simulink model "Power_system_RZA_tau"  (R2017a)
settings: Solver=ode45  StartTime=0.0  StopTime=150  MaxStep=1e-4  RelTol=1e-3
values from neighbouring files (symbols this model uses):
  A2 = [0 1;0 0]    [Power_system_RZA_m.m]
  alpha = [alpha1;alpha0]    [Power_system_RZA_m.m]
  alpha0 = 1    [Power_system_RZA_m.m]
  B2 = [0;1]    [Power_system_RZA_m.m]
  C2 = [1 0]    [Power_system_RZA_m.m]
  Delta_f0 = 0    [Power_system_RZA_m.m]
  Delta_P0 = 0    [Power_system_RZA_m.m]
  Delta_X0 = 0.011    [Power_system_RZA_m.m]
  denC = conv([1 0],[tauC 1])    [Power_system_RZA_m.m]
  gn = -2*Klm/Tlm/Tg    (= -1.66666666667)    [Power_system_RZA_m.m]
  Gn = 3/Thn/Klm*(-1-Tlm/Thn)    (= -1.875)    [Power_system_RZA_m.m]
  Klm = 1    [Power_system_RZA_m.m]
  ks = -10    [Power_system_RZA_m.m]
  numC = [1.8124 -18.8558 0.1523]    [Power_system_RZA_m.m]
  ooverline_sat = overline_sat -1/ks    (= 20000.1)    [Power_system_RZA_m.m]
  overline_phin = [phin2; phin1]    [Power_system_RZA_m.m]
  overline_sat = 20000    [Power_system_RZA_m.m]
  psin = Klm/Tlm/Thn + Klm/Tlm/Tg    (= 0.875)    [Power_system_RZA_m.m]
  R = 0.05    [Power_system_RZA_m.m]
  Sn = 1/Thn    (= 0.25)    [Power_system_RZA_m.m]
  tau = 0.001    [Power_system_RZA_m.m]
  tau1 = 0.05    [Power_system_RZA_m.m]
  tau2 = 0.005    [Power_system_RZA_m.m]
  tau3 = 0.001    [Power_system_RZA_m.m]
  Tg = 0.2    [Power_system_RZA_m.m]
  Th2 = 6    [Power_system_RZA_m.m]
  Tlm = 6    [Power_system_RZA_m.m]
  ttrig = 60    [Power_system_RZA_m.m]
  underline_Delta1 = [tau1 0;0 tau1^2]    [Power_system_RZA_m.m]
  underline_Delta2 = [tau2 0;0 tau2^2]    [Power_system_RZA_m.m]
  underline_Delta3 = [tau3 0;0 tau3^2]    [Power_system_RZA_m.m]
  uunderline_sat = underline_sat + 1/ks    (= -20000.1)    [Power_system_RZA_m.m]
  zna0 = -0.001    [Power_system_RZA_m.m]
settings Model: Creator=Gyunghoon  LastModifiedBy=Gyunghoon
settings DataIOCC: LimitDataPoints=on  SaveFormat=Array
settings OptimizationCC: BlockReduction=off  BooleanDataType=off  LifeSpan=inf
settings DebuggingCC: SaveWithParameterizedLinksMsg=none  UnderspecifiedInitializationDetection=Classic  MergeDetectMultiDrivingBlocksExec=none  SignalResolutionControl=TryResolveAllWithWarning  SFUnexpectedBacktrackingDiag=warning  SFNoUnconditionalDefaultTransitionDiag=warning  SFExecutionAtInitializationDiag=none
settings HardwareCC: ProdBitPerPointer=32  ProdBitPerSizeT=32  ProdBitPerPtrDiffT=32  ProdLargestAtomicFloat=None  ProdIntDivRoundTo=Undefined  ProdEndianess=Unspecified  ProdWordSize=32  ProdHWDeviceType=32-bit Generic  TargetUnknown=on
settings ModelReferenceCC: PropagateSignalLabelsOutOfModel=off
settings GRTTargetCC: TargetLangStandard=C89/C90 (ANSI)  GeneratePreprocessorConditionals=Disable all
settings ConfigComp: CovMetricSettings=dw  CovHtmlReporting=on  CovSaveCumulativeToWorkspaceVar=on  CovSaveSingleToWorkspaceVar=on  CovExternalEMLEnable=off  CovSFcnEnable=off

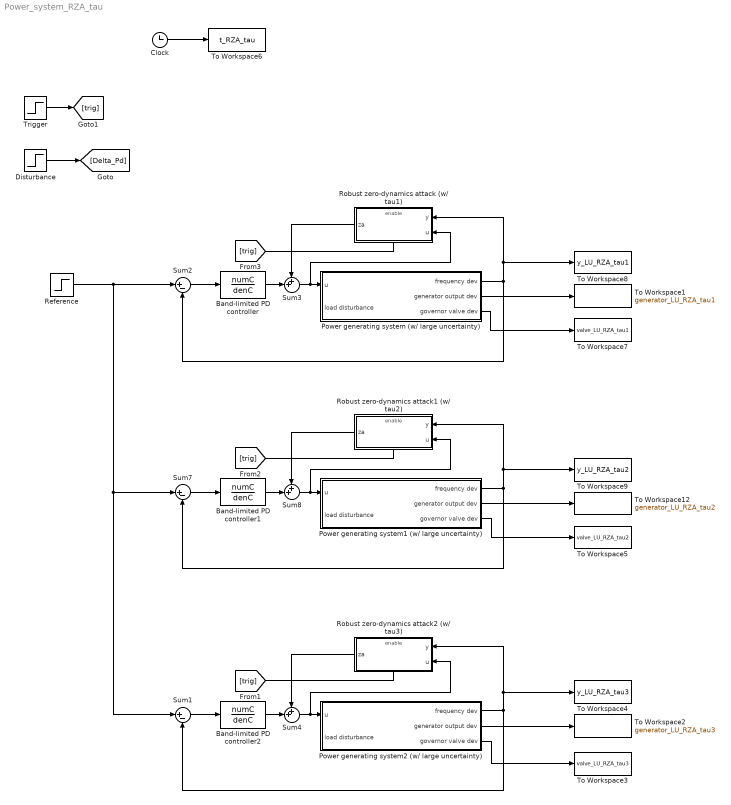
== system Power_system_RZA_tau ==
  Band-limited PD controller : TransferFcn  Numerator=numC  Denominator=denC
  Band-limited PD controller1 : TransferFcn  Numerator=numC  Denominator=denC
  Band-limited PD controller2 : TransferFcn  Numerator=numC  Denominator=denC
  Clock : Clock
  Disturbance : Step  Time=0  After=0.01  SampleTime=0
  Power generating system (w/ large uncertainty) : Subsystem
  Power generating system1 (w/ large uncertainty) : Subsystem
  Power generating system2 (w/ large uncertainty) : Subsystem
  Reference : Step  Time=0  After=0  SampleTime=0
  Robust zero-dynamics attack (w/ tau1) : Subsystem  TreatAsAtomicUnit=on
  Robust zero-dynamics attack1 (w/ tau2) : Subsystem  TreatAsAtomicUnit=on
  Robust zero-dynamics attack2 (w/ tau3) : Subsystem  TreatAsAtomicUnit=on
  Sum1 : Sum  Inputs=|+-
  Sum2 : Sum  Inputs=|+-
  Sum3 : Sum  Inputs=++|
  Sum4 : Sum  Inputs=++|
  Sum7 : Sum  Inputs=|+-
  Sum8 : Sum  Inputs=++|
  To Workspace1 : ToWorkspace  VariableName=generator_LU_RZA_tau1  SampleTime=-1
  To Workspace12 : ToWorkspace  VariableName=generator_LU_RZA_tau2  SampleTime=-1
  To Workspace2 : ToWorkspace  VariableName=generator_LU_RZA_tau3  SampleTime=-1
  To Workspace3 : ToWorkspace  VariableName=valve_LU_RZA_tau3  SampleTime=-1
  To Workspace4 : ToWorkspace  VariableName=y_LU_RZA_tau3  SampleTime=-1
  To Workspace5 : ToWorkspace  VariableName=valve_LU_RZA_tau2  SampleTime=-1
  To Workspace6 : ToWorkspace  VariableName=t_RZA_tau  SampleTime=-1
  To Workspace7 : ToWorkspace  VariableName=valve_LU_RZA_tau1  SampleTime=-1
  To Workspace8 : ToWorkspace  VariableName=y_LU_RZA_tau1  SampleTime=-1
  To Workspace9 : ToWorkspace  VariableName=y_LU_RZA_tau2  SampleTime=-1
  Trigger : Step  Time=ttrig  SampleTime=0
  wires:
  Disturbance/1 -> [Delta_Pd]
  Sum7/1 -> Band-limited PD controller1/1
  Band-limited PD controller1/1 -> Sum8/2
  Power generating system1 (w/ large uncertainty)/3(governor valve dev) -> To Workspace5/1
  Clock/1 -> To Workspace6/1
  Power generating system1 (w/ large uncertainty)/1(frequency dev) -> To Workspace9/1, Robust zero-dynamics attack1 (w/ tau2)/1(y), Sum7/2
  Sum8/1 -> Robust zero-dynamics attack1 (w/ tau2)/2(u), Power generating system1 (w/ large uncertainty)/1(u)
  Robust zero-dynamics attack1 (w/ tau2)/1(za) -> Sum8/1
  Trigger/1 -> [trig]
  [trig] -> Robust zero-dynamics attack1 (w/ tau2)/Enable
  Power generating system1 (w/ large uncertainty)/2(generator output dev) -> To Workspace12/1
  Sum1/1 -> Band-limited PD controller2/1
  Band-limited PD controller2/1 -> Sum4/2
  Power generating system2 (w/ large uncertainty)/3(governor valve dev) -> To Workspace3/1
  Power generating system2 (w/ large uncertainty)/1(frequency dev) -> To Workspace4/1, Robust zero-dynamics attack2 (w/ tau3)/1(y), Sum1/2
  Sum4/1 -> Robust zero-dynamics attack2 (w/ tau3)/2(u), Power generating system2 (w/ large uncertainty)/1(u)
  Robust zero-dynamics attack2 (w/ tau3)/1(za) -> Sum4/1
  [trig] -> Robust zero-dynamics attack2 (w/ tau3)/Enable
  Power generating system2 (w/ large uncertainty)/2(generator output dev) -> To Workspace2/1
  Sum2/1 -> Band-limited PD controller/1
  Reference/1 -> Sum1/1, Sum7/1, Sum2/1
  Band-limited PD controller/1 -> Sum3/2
  Power generating system (w/ large uncertainty)/3(governor valve dev) -> To Workspace7/1
  Power generating system (w/ large uncertainty)/1(frequency dev) -> To Workspace8/1, Robust zero-dynamics attack (w/ tau1)/1(y), Sum2/2
  Sum3/1 -> Robust zero-dynamics attack (w/ tau1)/2(u), Power generating system (w/ large uncertainty)/1(u)
  Robust zero-dynamics attack (w/ tau1)/1(za) -> Sum3/1
  [trig] -> Robust zero-dynamics attack (w/ tau1)/Enable
  Power generating system (w/ large uncertainty)/2(generator output dev) -> To Workspace1/1

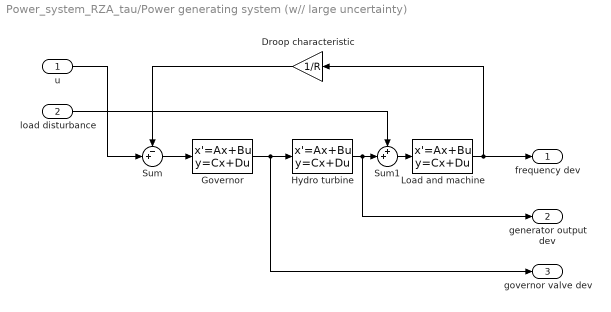
== system Power_system_RZA_tau/Power generating system (w// large uncertainty) ==
  u : Inport
  load disturbance : Inport  Port=2
  Droop characteristic : Gain  Gain=1/R
  Governor : StateSpace  A=-1/Tg  B=1/Tg  D=0  X0=Delta_X0
  Hydro turbine : StateSpace  A=-2/Th2  B=6/Th2  D=-2  X0=Delta_P0+2*Delta_X0
  Load and machine : StateSpace  A=-1/Tlm  B=Klm/Tlm  D=0  X0=Delta_f0
  Sum : Sum  Inputs=-+|
  Sum1 : Sum  Inputs=++|
  frequency dev : Outport
  generator output dev : Outport  Port=2
  governor valve dev : Outport  Port=3
  wires:
  u/1 -> Sum/2
  Droop characteristic/1 -> Sum/1
  Load and machine/1 -> Droop characteristic/1, frequency dev/1
  Hydro turbine/1 -> generator output dev/1, Sum1/2
  Sum/1 -> Governor/1
  Governor/1 -> Hydro turbine/1, governor valve dev/1
  Sum1/1 -> Load and machine/1
  load disturbance/1 -> Sum1/1

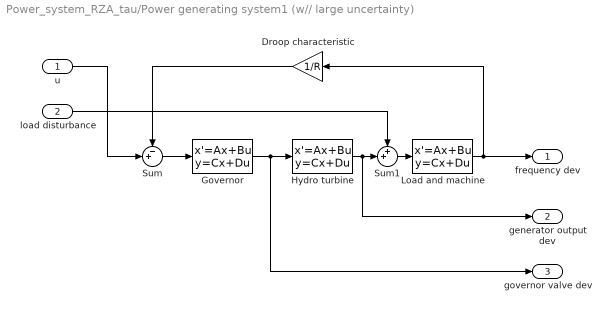
== system Power_system_RZA_tau/Power generating system1 (w// large uncertainty) ==
  u : Inport
  load disturbance : Inport  Port=2
  Droop characteristic : Gain  Gain=1/R
  Governor : StateSpace  A=-1/Tg  B=1/Tg  D=0  X0=Delta_X0
  Hydro turbine : StateSpace  A=-2/Th2  B=6/Th2  D=-2  X0=Delta_P0+2*Delta_X0
  Load and machine : StateSpace  A=-1/Tlm  B=Klm/Tlm  D=0  X0=Delta_f0
  Sum : Sum  Inputs=-+|
  Sum1 : Sum  Inputs=++|
  frequency dev : Outport
  generator output dev : Outport  Port=2
  governor valve dev : Outport  Port=3
  wires:
  u/1 -> Sum/2
  Droop characteristic/1 -> Sum/1
  Load and machine/1 -> Droop characteristic/1, frequency dev/1
  Hydro turbine/1 -> generator output dev/1, Sum1/2
  Sum/1 -> Governor/1
  Governor/1 -> Hydro turbine/1, governor valve dev/1
  Sum1/1 -> Load and machine/1
  load disturbance/1 -> Sum1/1

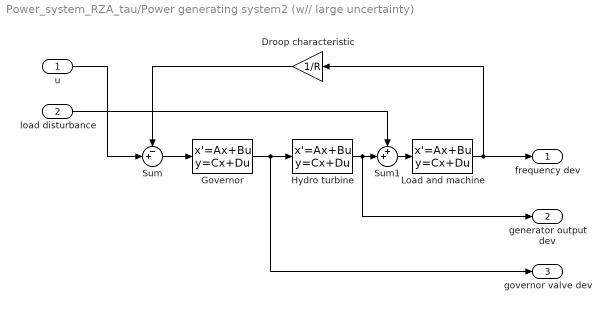
== system Power_system_RZA_tau/Power generating system2 (w// large uncertainty) ==
  u : Inport
  load disturbance : Inport  Port=2
  Droop characteristic : Gain  Gain=1/R
  Governor : StateSpace  A=-1/Tg  B=1/Tg  D=0  X0=Delta_X0
  Hydro turbine : StateSpace  A=-2/Th2  B=6/Th2  D=-2  X0=Delta_P0+2*Delta_X0
  Load and machine : StateSpace  A=-1/Tlm  B=Klm/Tlm  D=0  X0=Delta_f0
  Sum : Sum  Inputs=-+|
  Sum1 : Sum  Inputs=++|
  frequency dev : Outport
  generator output dev : Outport  Port=2
  governor valve dev : Outport  Port=3
  wires:
  u/1 -> Sum/2
  Droop characteristic/1 -> Sum/1
  Load and machine/1 -> Droop characteristic/1, frequency dev/1
  Hydro turbine/1 -> generator output dev/1, Sum1/2
  Sum/1 -> Governor/1
  Governor/1 -> Hydro turbine/1, governor valve dev/1
  Sum1/1 -> Load and machine/1
  load disturbance/1 -> Sum1/1

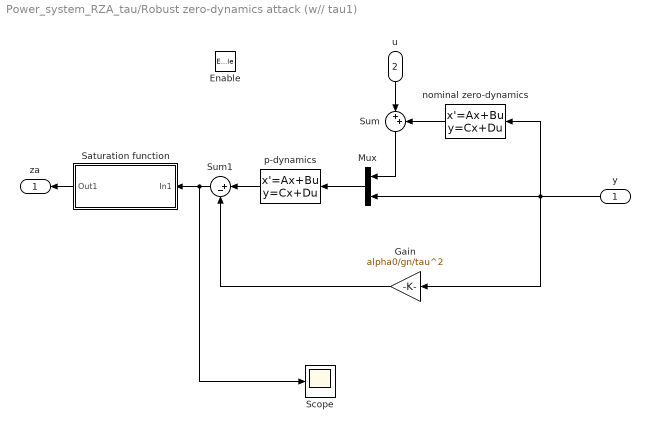
== system Power_system_RZA_tau/Robust zero-dynamics attack (w// tau1) ==
  y : Inport
  u : Inport  Port=2
  Enable : EnablePort  PropagateVarSize=During execution
  "\tSaturation function" : Subsystem
  Gain : Gain  Gain=alpha0/gn/tau^2
  Mux : Mux  Inputs=2
  Scope : Scope
  Sum : Sum  Inputs=|++
  Sum1 : Sum  Inputs=|+-
  nominal zero-dynamics : StateSpace  A=Sn  B=Gn  C=psin/gn  D=0  X0=zna0
  p-dynamics : StateSpace  A=A2-inv(underline_Delta1)*alpha*C2  B=[alpha0/tau1^2*B2 alpha0/tau1^2/gn*(overline_phin+inv(underline_Delta1)*alpha)]  C=C2  D=[0 0]  X0=[0 0]
  za : Outport  OutputWhenDisabled=reset  InitialOutput=0
  wires:
  y/1 -> nominal zero-dynamics/1, Gain/1, Mux/2
  "\tSaturation function"/1(Out1) -> za/1
  Mux/1 -> p-dynamics/1
  u/1 -> Sum/1
  nominal zero-dynamics/1 -> Sum/2
  Sum/1 -> Mux/1
  p-dynamics/1 -> Sum1/1
  Sum1/1 -> "\tSaturation function"/1(In1), Scope/1
  Gain/1 -> Sum1/2

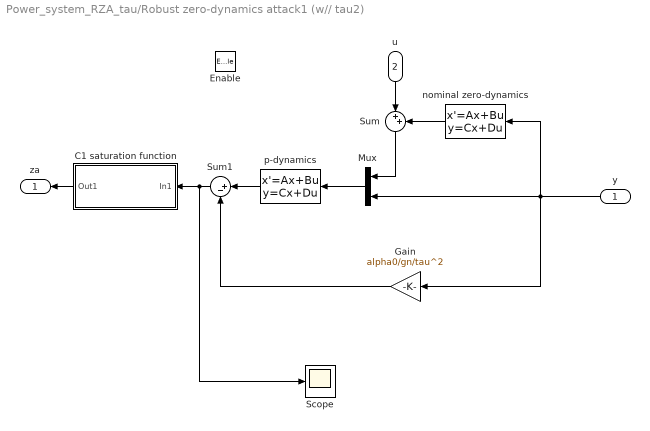
== system Power_system_RZA_tau/Robust zero-dynamics attack1 (w// tau2) ==
  y : Inport
  u : Inport  Port=2
  Enable : EnablePort  PropagateVarSize=During execution
  C1 saturation function : Subsystem
  Gain : Gain  Gain=alpha0/gn/tau^2
  Mux : Mux  Inputs=2
  Scope : Scope
  Sum : Sum  Inputs=|++
  Sum1 : Sum  Inputs=|+-
  nominal zero-dynamics : StateSpace  A=Sn  B=Gn  C=psin/gn  D=0  X0=zna0
  p-dynamics : StateSpace  A=A2-inv(underline_Delta2)*alpha*C2  B=[alpha0/tau2^2*B2 alpha0/tau2^2/gn*(overline_phin+inv(underline_Delta2)*alpha)]  C=C2  D=[0 0]  X0=[0 0]
  za : Outport  OutputWhenDisabled=reset  InitialOutput=0
  wires:
  y/1 -> nominal zero-dynamics/1, Gain/1, Mux/2
  C1 saturation function/1(Out1) -> za/1
  Mux/1 -> p-dynamics/1
  u/1 -> Sum/1
  nominal zero-dynamics/1 -> Sum/2
  Sum/1 -> Mux/1
  p-dynamics/1 -> Sum1/1
  Sum1/1 -> C1 saturation function/1(In1), Scope/1
  Gain/1 -> Sum1/2

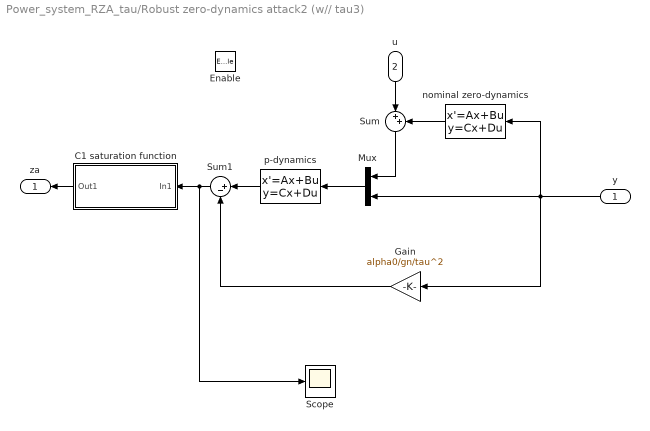
== system Power_system_RZA_tau/Robust zero-dynamics attack2 (w// tau3) ==
  y : Inport
  u : Inport  Port=2
  Enable : EnablePort  PropagateVarSize=During execution
  C1 saturation function : Subsystem
  Gain : Gain  Gain=alpha0/gn/tau^2
  Mux : Mux  Inputs=2
  Scope : Scope
  Sum : Sum  Inputs=|++
  Sum1 : Sum  Inputs=|+-
  nominal zero-dynamics : StateSpace  A=Sn  B=Gn  C=psin/gn  D=0  X0=zna0
  p-dynamics : StateSpace  A=A2-inv(underline_Delta3)*alpha*C2  B=[alpha0/tau3^2*B2 alpha0/tau3^2/gn*(overline_phin+inv(underline_Delta3)*alpha)]  C=C2  D=[0 0]  X0=[0 0]
  za : Outport  OutputWhenDisabled=reset  InitialOutput=0
  wires:
  y/1 -> nominal zero-dynamics/1, Gain/1, Mux/2
  C1 saturation function/1(Out1) -> za/1
  Mux/1 -> p-dynamics/1
  u/1 -> Sum/1
  nominal zero-dynamics/1 -> Sum/2
  Sum/1 -> Mux/1
  p-dynamics/1 -> Sum1/1
  Sum1/1 -> C1 saturation function/1(In1), Scope/1
  Gain/1 -> Sum1/2

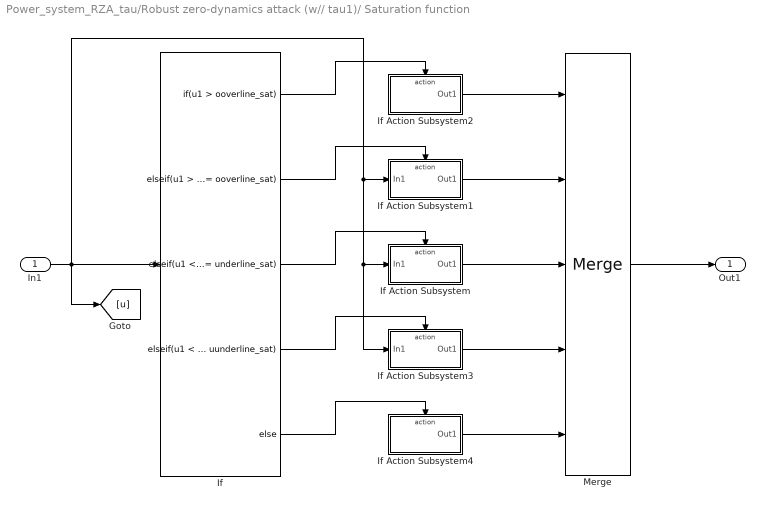
== system Power_system_RZA_tau/Robust zero-dynamics attack (w// tau1)/	Saturation function ==
  In1 : Inport
  If : If  IfExpression=u1 > ooverline_sat  ElseIfExpressions=u1 > overline_sat & u1 <= ooverline_sat, u1 <= overline_sat & u1>= underline_sat, u1 < underline_sat & u1 >= uunderline_sat
  If Action Subsystem : Subsystem  TreatAsAtomicUnit=on
  If Action Subsystem1 : Subsystem  TreatAsAtomicUnit=on
  If Action Subsystem2 : Subsystem  TreatAsAtomicUnit=on
  If Action Subsystem3 : Subsystem  TreatAsAtomicUnit=on
  If Action Subsystem4 : Subsystem  TreatAsAtomicUnit=on
  Merge : Merge  Inputs=5
  Out1 : Outport
  wires:
  In1/1 -> If Action Subsystem3/1(In1), If Action Subsystem/1(In1), If Action Subsystem1/1(In1), [u], If/1
  Merge/1 -> Out1/1
  If/3 -> If Action Subsystem/Action
  If Action Subsystem/1(Out1) -> Merge/3
  If/2 -> If Action Subsystem1/Action
  If Action Subsystem2/1(Out1) -> Merge/1
  If/1 -> If Action Subsystem2/Action
  If Action Subsystem3/1(Out1) -> Merge/4
  If/4 -> If Action Subsystem3/Action
  If Action Subsystem4/1(Out1) -> Merge/5
  If/5 -> If Action Subsystem4/Action
  If Action Subsystem1/1(Out1) -> Merge/2

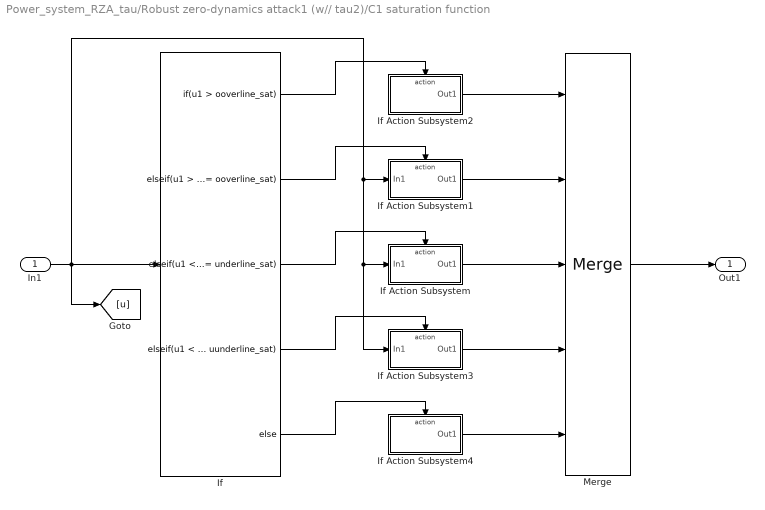
== system Power_system_RZA_tau/Robust zero-dynamics attack1 (w// tau2)/C1 saturation function ==
  In1 : Inport
  If : If  IfExpression=u1 > ooverline_sat  ElseIfExpressions=u1 > overline_sat & u1 <= ooverline_sat, u1 <= overline_sat & u1>= underline_sat, u1 < underline_sat & u1 >= uunderline_sat
  If Action Subsystem : Subsystem  TreatAsAtomicUnit=on
  If Action Subsystem1 : Subsystem  TreatAsAtomicUnit=on
  If Action Subsystem2 : Subsystem  TreatAsAtomicUnit=on
  If Action Subsystem3 : Subsystem  TreatAsAtomicUnit=on
  If Action Subsystem4 : Subsystem  TreatAsAtomicUnit=on
  Merge : Merge  Inputs=5
  Out1 : Outport
  wires:
  In1/1 -> If Action Subsystem3/1(In1), If Action Subsystem/1(In1), If Action Subsystem1/1(In1), [u], If/1
  Merge/1 -> Out1/1
  If/3 -> If Action Subsystem/Action
  If Action Subsystem/1(Out1) -> Merge/3
  If/2 -> If Action Subsystem1/Action
  If Action Subsystem2/1(Out1) -> Merge/1
  If/1 -> If Action Subsystem2/Action
  If Action Subsystem3/1(Out1) -> Merge/4
  If/4 -> If Action Subsystem3/Action
  If Action Subsystem4/1(Out1) -> Merge/5
  If/5 -> If Action Subsystem4/Action
  If Action Subsystem1/1(Out1) -> Merge/2

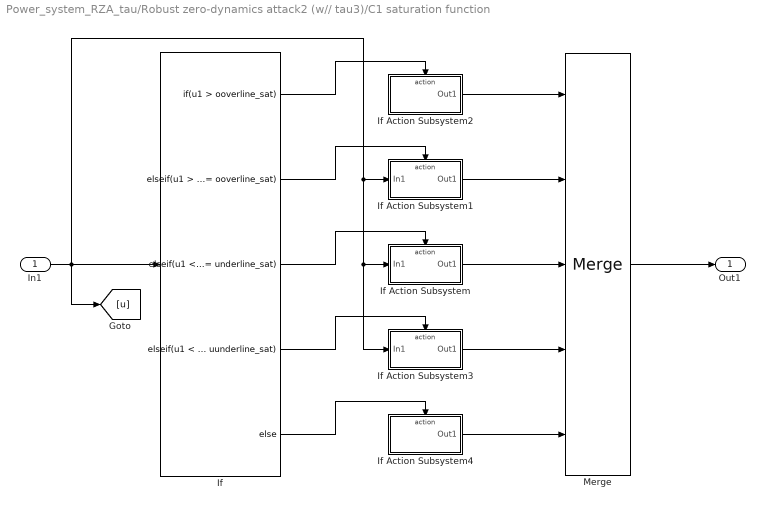
== system Power_system_RZA_tau/Robust zero-dynamics attack2 (w// tau3)/C1 saturation function ==
  In1 : Inport
  If : If  IfExpression=u1 > ooverline_sat  ElseIfExpressions=u1 > overline_sat & u1 <= ooverline_sat, u1 <= overline_sat & u1>= underline_sat, u1 < underline_sat & u1 >= uunderline_sat
  If Action Subsystem : Subsystem  TreatAsAtomicUnit=on
  If Action Subsystem1 : Subsystem  TreatAsAtomicUnit=on
  If Action Subsystem2 : Subsystem  TreatAsAtomicUnit=on
  If Action Subsystem3 : Subsystem  TreatAsAtomicUnit=on
  If Action Subsystem4 : Subsystem  TreatAsAtomicUnit=on
  Merge : Merge  Inputs=5
  Out1 : Outport
  wires:
  In1/1 -> If Action Subsystem3/1(In1), If Action Subsystem/1(In1), If Action Subsystem1/1(In1), [u], If/1
  Merge/1 -> Out1/1
  If/3 -> If Action Subsystem/Action
  If Action Subsystem/1(Out1) -> Merge/3
  If/2 -> If Action Subsystem1/Action
  If Action Subsystem2/1(Out1) -> Merge/1
  If/1 -> If Action Subsystem2/Action
  If Action Subsystem3/1(Out1) -> Merge/4
  If/4 -> If Action Subsystem3/Action
  If Action Subsystem4/1(Out1) -> Merge/5
  If/5 -> If Action Subsystem4/Action
  If Action Subsystem1/1(Out1) -> Merge/2

== system Power_system_RZA_tau/Robust zero-dynamics attack (w// tau1)/	Saturation function/If Action Subsystem ==
  In1 : Inport
  Action Port : ActionPort  ActionType=elseif
  Out1 : Outport
  wires:
  In1/1 -> Out1/1

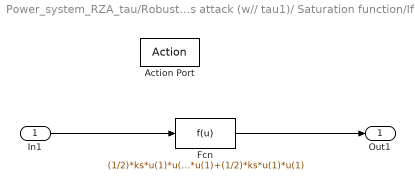
== system Power_system_RZA_tau/Robust zero-dynamics attack (w// tau1)/	Saturation function/If Action Subsystem1 ==
  In1 : Inport
  Action Port : ActionPort  ActionType=elseif
  Fcn : Fcn  Expr=(1/2)*ks*u(1)*u(1)+(-ks*overline_sat+1)*u(1)+(1/2)*ks*u(1)*u(1)
  Out1 : Outport
  wires:
  Fcn/1 -> Out1/1
  In1/1 -> Fcn/1

== system Power_system_RZA_tau/Robust zero-dynamics attack (w// tau1)/	Saturation function/If Action Subsystem2 ==
  Action Port : ActionPort  ActionType=then
  Constant : Constant  Value=ooverline_sat
  Out1 : Outport
  wires:
  Constant/1 -> Out1/1

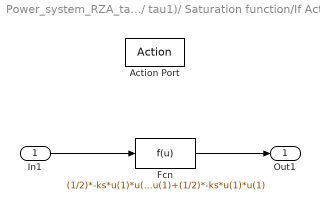
== system Power_system_RZA_tau/Robust zero-dynamics attack (w// tau1)/	Saturation function/If Action Subsystem3 ==
  In1 : Inport
  Action Port : ActionPort  ActionType=elseif
  Fcn : Fcn  Expr=(1/2)*-ks*u(1)*u(1)+(ks*overline_sat+1)*u(1)+(1/2)*-ks*u(1)*u(1)
  Out1 : Outport
  wires:
  Fcn/1 -> Out1/1
  In1/1 -> Fcn/1

== system Power_system_RZA_tau/Robust zero-dynamics attack (w// tau1)/	Saturation function/If Action Subsystem4 ==
  Action Port : ActionPort  ActionType=else
  Constant : Constant  Value=[uunderline_sat]
  Out1 : Outport
  wires:
  Constant/1 -> Out1/1

== system Power_system_RZA_tau/Robust zero-dynamics attack1 (w// tau2)/C1 saturation function/If Action Subsystem ==
  In1 : Inport
  Action Port : ActionPort  ActionType=elseif
  Out1 : Outport
  wires:
  In1/1 -> Out1/1

== system Power_system_RZA_tau/Robust zero-dynamics attack1 (w// tau2)/C1 saturation function/If Action Subsystem1 ==
  In1 : Inport
  Action Port : ActionPort  ActionType=elseif
  Fcn : Fcn  Expr=(1/2)*ks*u(1)*u(1)+(-ks*overline_sat+1)*u(1)+(1/2)*ks*u(1)*u(1)
  Out1 : Outport
  wires:
  Fcn/1 -> Out1/1
  In1/1 -> Fcn/1

== system Power_system_RZA_tau/Robust zero-dynamics attack1 (w// tau2)/C1 saturation function/If Action Subsystem2 ==
  Action Port : ActionPort  ActionType=then
  Constant : Constant  Value=ooverline_sat
  Out1 : Outport
  wires:
  Constant/1 -> Out1/1

== system Power_system_RZA_tau/Robust zero-dynamics attack1 (w// tau2)/C1 saturation function/If Action Subsystem3 ==
  In1 : Inport
  Action Port : ActionPort  ActionType=elseif
  Fcn : Fcn  Expr=(1/2)*-ks*u(1)*u(1)+(ks*overline_sat+1)*u(1)+(1/2)*-ks*u(1)*u(1)
  Out1 : Outport
  wires:
  Fcn/1 -> Out1/1
  In1/1 -> Fcn/1

== system Power_system_RZA_tau/Robust zero-dynamics attack1 (w// tau2)/C1 saturation function/If Action Subsystem4 ==
  Action Port : ActionPort  ActionType=else
  Constant : Constant  Value=[uunderline_sat]
  Out1 : Outport
  wires:
  Constant/1 -> Out1/1

== system Power_system_RZA_tau/Robust zero-dynamics attack2 (w// tau3)/C1 saturation function/If Action Subsystem ==
  In1 : Inport
  Action Port : ActionPort  ActionType=elseif
  Out1 : Outport
  wires:
  In1/1 -> Out1/1

== system Power_system_RZA_tau/Robust zero-dynamics attack2 (w// tau3)/C1 saturation function/If Action Subsystem1 ==
  In1 : Inport
  Action Port : ActionPort  ActionType=elseif
  Fcn : Fcn  Expr=(1/2)*ks*u(1)*u(1)+(-ks*overline_sat+1)*u(1)+(1/2)*ks*u(1)*u(1)
  Out1 : Outport
  wires:
  Fcn/1 -> Out1/1
  In1/1 -> Fcn/1

== system Power_system_RZA_tau/Robust zero-dynamics attack2 (w// tau3)/C1 saturation function/If Action Subsystem2 ==
  Action Port : ActionPort  ActionType=then
  Constant : Constant  Value=ooverline_sat
  Out1 : Outport
  wires:
  Constant/1 -> Out1/1

== system Power_system_RZA_tau/Robust zero-dynamics attack2 (w// tau3)/C1 saturation function/If Action Subsystem3 ==
  In1 : Inport
  Action Port : ActionPort  ActionType=elseif
  Fcn : Fcn  Expr=(1/2)*-ks*u(1)*u(1)+(ks*overline_sat+1)*u(1)+(1/2)*-ks*u(1)*u(1)
  Out1 : Outport
  wires:
  Fcn/1 -> Out1/1
  In1/1 -> Fcn/1

== system Power_system_RZA_tau/Robust zero-dynamics attack2 (w// tau3)/C1 saturation function/If Action Subsystem4 ==
  Action Port : ActionPort  ActionType=else
  Constant : Constant  Value=[uunderline_sat]
  Out1 : Outport
  wires:
  Constant/1 -> Out1/1
